simulink model "modelo_psub_2022"  (R2025a)
settings: Solver=VariableStepAuto  StartTime=0.0  StopTime=10.0  RelTol=1e-3
libraries: simulink x3
settings Model: Creator=joaof  LastModifiedBy=joaof

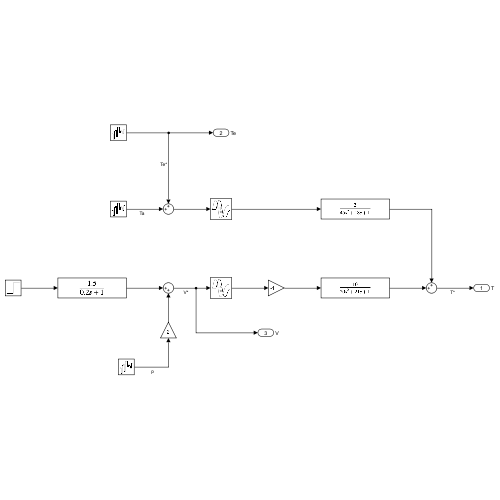
[thumbnail: Simulink's stored preview of the top-level diagram]
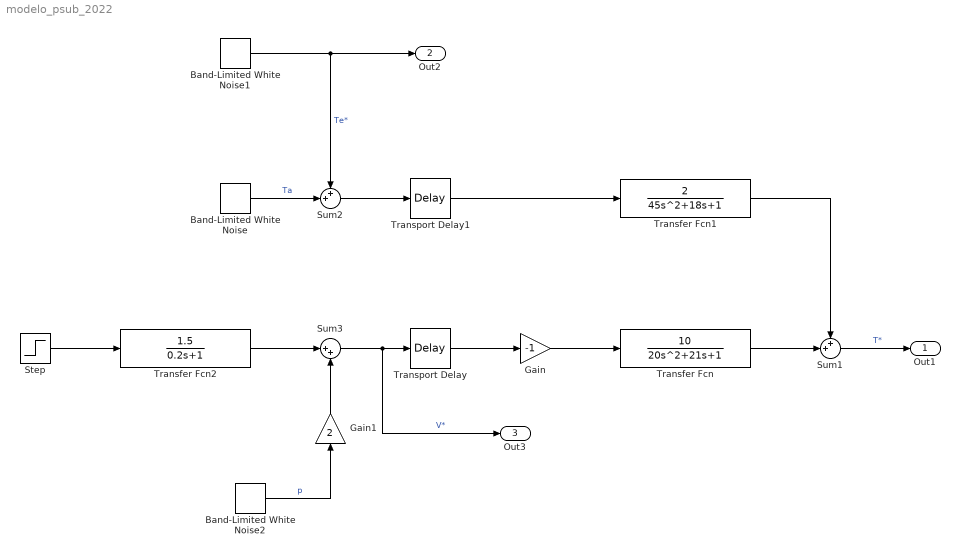
== system modelo_psub_2022 ==
  Band-Limited White Noise : simulink/Sources/Band-Limited White Noise  Cov=[0.1]  Ts=0.1  seed=[23341]
  Band-Limited White Noise1 : simulink/Sources/Band-Limited White Noise  Cov=[0.1]  Ts=0.1  seed=[23341]
  Band-Limited White Noise2 : simulink/Sources/Band-Limited White Noise  Cov=[0.1]  Ts=0.1  seed=[23341]
  Gain : Gain  Gain=-1
  Gain1 : Gain  Gain=2
  Step : Step  SampleTime=0
  Sum1 : Sum  Inputs=++|
  Sum2 : Sum  Inputs=++|
  Sum3 : Sum  Inputs=|++
  Transfer Fcn : TransferFcn  Numerator=[10]  Denominator=[20 21 1]
  Transfer Fcn1 : TransferFcn  Numerator=[2]  Denominator=[45 18 1]
  Transfer Fcn2 : TransferFcn  Numerator=[1.5]  Denominator=[0.2 1]
  Transport Delay : TransportDelay  DelayTime=40
  Transport Delay1 : TransportDelay  DelayTime=40
  Out1 : Outport  SignalName=T
  Out2 : Outport  Port=2  SignalName=Te
  Out3 : Outport  Port=3  SignalName=V
  wires:
  Transport Delay/1 -> Gain/1
  Gain/1 -> Transfer Fcn/1
  Transport Delay1/1 -> Transfer Fcn1/1
  Sum2/1 -> Transport Delay1/1
  Band-Limited White Noise1/1 -> Out2/1, Sum2/1  "Te*"
  Band-Limited White Noise/1 -> Sum2/2  "Ta"
  Sum3/1 -> Out3/1, Transport Delay/1  "V*"
  Transfer Fcn/1 -> Sum1/2
  Transfer Fcn1/1 -> Sum1/1
  Transfer Fcn2/1 -> Sum3/1
  Band-Limited White Noise2/1 -> Gain1/1  "p"
  Gain1/1 -> Sum3/2
  Step/1 -> Transfer Fcn2/1
  Sum1/1 -> Out1/1  "T*"
